simulink model "ECM_EKF_WLTP_kalman"  (R2021b)
settings: Solver=FixedStepDiscrete  StartTime=0.0  StopTime=100000  FixedStep=Ts_data  RelTol=1e-3
PreLoadFcn:
  | % PreLoadFcn — add repo root to MATLAB path before model loads
  | try
  |     mdlName = bdroot;
  |     mdlFile = get_param(mdlName,'FileName');
  |     mdlDir  = fileparts(mdlFile);
  |     repoRoot = fileparts(mdlDir);
  | 
  | 
  |     addpath(genpath(repoRoot));
  |     cd(repoRoot);   % ensure relative paths work while loading
  | catch ME
  |     warning('PreLoadFcn path init failed: %s', ME.message);
  | end
PostLoadFcn:
  | % LoadFcn — run scripts after model loads
  | try
  |     setup_ecm;               % 1) create/overwrite data dictionary with LUTs
  |     setup_ekf;               % 2) upsert EKF params into dictionary
  |     Measured_data_import;    % 3) import measured data to base workspace
  |     fprintf('[%s] Auto-init complete.\n', bdroot);
  | catch ME
  |     warning('LoadFcn auto-init failed: %s', ME.message);
  | end
undefined symbols (not defined in the file or in its folder): C1_lut, C2_lut, crate_bp, DiscIntNeverNeededParam, H_min, OCV_dVoc_dSOC, OCV_lut, OCV_SOC_bp, Q_proc, R0_lut, R1_lut, R2_lut, R_meas, SoC0_guess, soc_bp, Ts_data
settings Model: DataDictionary=ecm_dd.sldd  Creator=ahmeds28  LastModifiedBy=ahmeds28

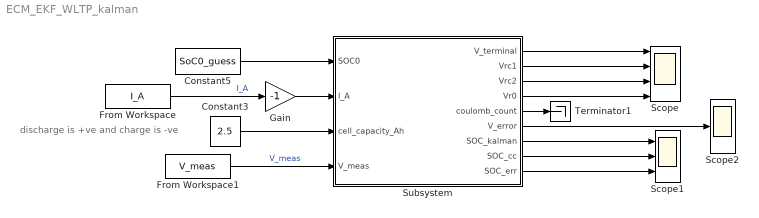
== system ECM_EKF_WLTP_kalman ==
  note: discharge is +ve and charge is -ve
  Constant3 : Constant  Value=2.5
  Constant5 : Constant  Value=SoC0_guess
  From Workspace : FromWorkspace  VariableName=I_A
  From Workspace1 : FromWorkspace  VariableName=V_meas
  Gain : Gain  Gain=-1
  Scope : Scope  NumInputPorts=4
  Scope1 : Scope  NumInputPorts=3
  Scope2 : Scope
  Subsystem : Subsystem
  Terminator1 : Terminator
  wires:
  Constant3/1 -> Subsystem/3(cell_capacity_Ah)
  From Workspace/1 -> Gain/1  "I_A"
  Constant5/1 -> Subsystem/1(SOC0)
  Subsystem/1(V_terminal) -> Scope/1
  Gain/1 -> Subsystem/2(I_A)
  From Workspace1/1 -> Subsystem/4(V_meas)  "V_meas"
  Subsystem/2(Vrc1) -> Scope/2
  Subsystem/3(Vrc2) -> Scope/3
  Subsystem/4(Vr0) -> Scope/4
  Subsystem/7(SOC_kalman) -> Scope1/1
  Subsystem/8(SOC_cc) -> Scope1/2
  Subsystem/9(SOC_err) -> Scope1/3
  Subsystem/6(V_error) -> Scope2/1
  Subsystem/5(coulomb_count) -> Terminator1/1

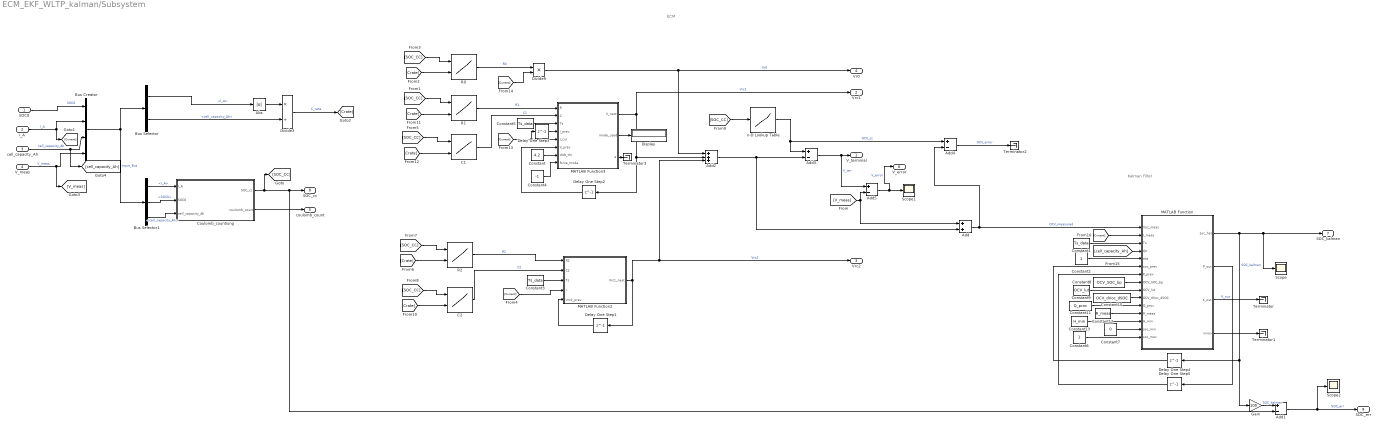
== system ECM_EKF_WLTP_kalman/Subsystem ==
  note: ECM
  note: Kalman Filter
  SOC0 : Inport
  I_A : Inport  Port=2
  cell_capacity_Ah : Inport  Port=3
  V_meas : Inport  Port=4
  Abs : Abs
  Add : Sum
  Add{1,3..5} (4 alike) : Sum  Inputs=+-
  Add2 : Sum  Inputs=+++
  Bus Creator : BusCreator  Inputs=4
  Bus Selector : BusSelector  OutputSignals=I_A,cell_capacity_Ah
  Bus Selector1 : BusSelector  OutputSignals=I_A,SOC0,cell_capacity_Ah
  C1 : Lookup_n-D  LookupTableObject=''  BreakpointsForDimension1=soc_bp  BreakpointsForDimension2=crate_bp  BreakpointsForDimension3=[5, 7]  BreakpointsForDimension1FirstPoint=10  BreakpointsForDimension2FirstPoint=10  BreakpointsForDimension1Spacing=12  BreakpointsForDimension2Spacing=12  IndexSearchMethod=Linear search  Table=C1_lut  InterpMethod=Flat  DiagnosticForOutOfRangeInput=Error  InternalRulePriority=Speed  RndMeth=Simplest  InputSameDT=on
      settings: InputPortMap=u0,u1
  C2 : Lookup_n-D  LookupTableObject=''  BreakpointsForDimension1=soc_bp  BreakpointsForDimension2=crate_bp  BreakpointsForDimension3=[5, 7]  BreakpointsForDimension1FirstPoint=10  BreakpointsForDimension2FirstPoint=10  BreakpointsForDimension1Spacing=12  BreakpointsForDimension2Spacing=12  IndexSearchMethod=Linear search  Table=C2_lut  InterpMethod=Flat  DiagnosticForOutOfRangeInput=Error  InternalRulePriority=Speed  RndMeth=Simplest  InputSameDT=on
      settings: InputPortMap=u0,u1
  Constant : Constant  Value=4.2
  Constant1 : Constant  Value=Ts_data
  Constant10 : Constant  Value=OCV_dVoc_dSOC
  Constant11 : Constant  Value=Q_proc
  Constant12 : Constant  Value=R_meas
  Constant13 : Constant  Value=H_min
  Constant2 : Constant
  Constant3 : Constant  Value=Ts_data
  Constant4 : Constant  Value=-1
  Constant5 : Constant  Value=Ts_data
  Constant6 : Constant
  Constant7 : Constant  Value=0
  Constant8 : Constant  Value=OCV_SOC_bp
  Constant9 : Constant  Value=OCV_lut
  Coulomb_countiung : Subsystem
  Delay One Step1 : Delay  DelayLength=1
  Delay One Step2 : Delay  DelayLength=1
  Delay One Step3 : Delay  DelayLength=1
  Delay One Step4 : Delay  DelayLength=1  InitialCondition=SoC0_guess/100
  Delay One Step5 : Delay  DelayLength=1  InitialCondition=0
  Display : Display
  Divide3 : Product  Inputs=*/
  Divide9 : Product  Inputs=**
  Gain : Gain  Gain=100
  MATLAB Function : MATLAB Function  TreatAsAtomicUnit=on
  MATLAB Function2 : MATLAB Function  TreatAsAtomicUnit=on
  MATLAB Function3 : MATLAB Function  TreatAsAtomicUnit=on
  R0 : Lookup_n-D  LookupTableObject=''  BreakpointsForDimension1=soc_bp  BreakpointsForDimension2=crate_bp  BreakpointsForDimension3=[5, 7]  BreakpointsForDimension1FirstPoint=10  BreakpointsForDimension2FirstPoint=10  BreakpointsForDimension1Spacing=12  BreakpointsForDimension2Spacing=12  IndexSearchMethod=Linear search  Table=R0_lut  InterpMethod=Flat  DiagnosticForOutOfRangeInput=Error  InternalRulePriority=Speed  RndMeth=Simplest  InputSameDT=on
      settings: InputPortMap=u0,u1
  R1 : Lookup_n-D  LookupTableObject=''  BreakpointsForDimension1=soc_bp  BreakpointsForDimension2=crate_bp  BreakpointsForDimension3=[5, 7]  BreakpointsForDimension1FirstPoint=10  BreakpointsForDimension2FirstPoint=10  BreakpointsForDimension1Spacing=12  BreakpointsForDimension2Spacing=12  IndexSearchMethod=Linear search  Table=R1_lut  InterpMethod=Flat  DiagnosticForOutOfRangeInput=Error  InternalRulePriority=Speed  RndMeth=Simplest  InputSameDT=on
      settings: InputPortMap=u0,u1
  R2 : Lookup_n-D  LookupTableObject=''  BreakpointsForDimension1=soc_bp  BreakpointsForDimension2=crate_bp  BreakpointsForDimension3=[5, 7]  BreakpointsForDimension1FirstPoint=10  BreakpointsForDimension2FirstPoint=10  BreakpointsForDimension1Spacing=12  BreakpointsForDimension2Spacing=12  IndexSearchMethod=Linear search  Table=R2_lut  InterpMethod=Flat  DiagnosticForOutOfRangeInput=Error  InternalRulePriority=Speed  RndMeth=Simplest  InputSameDT=on
      settings: InputPortMap=u0,u1
  Scope : Scope
  Scope1 : Scope
  Scope2 : Scope
  Terminator{,1..3} (4 alike) : Terminator
  n-D Lookup Table : Lookup_n-D  NumberOfTableDimensions=1  BreakpointsForDimension1=OCV_SOC_bp  BreakpointsForDimension3=[5, 7]  Table=OCV_lut  InternalRulePriority=Speed  RndMeth=Simplest  InputSameDT=on
  V_terminal : Outport
  Vrc1 : Outport  Port=2
  Vrc2 : Outport  Port=3
  Vr0 : Outport  Port=4
  coulomb_count : Outport  Port=5
  V_error : Outport  Port=6
  SOC_kalman : Outport  Port=7
  SOC_cc : Outport  Port=8
  SOC_err : Outport  Port=9
  wires:
  Bus Selector/1 -> Abs/1  "<I_A>"
  Bus Selector/2 -> Divide3/2  "<cell_capacity_Ah>"
  Divide3/1 -> [Crate]  "C_rate"
  Abs/1 -> Divide3/1
  [Crate] -> R0/2
  [SOC_CC] -> R0/1
  [Crate] -> R2/2
  [SOC_CC] -> R2/1
  [Crate] -> C2/2
  [SOC_CC] -> C2/1
  R0/1 -> Divide9/1  "R0"
  [Current] -> Divide9/2
  Divide9/1 -> Vr0/1, Add2/1  "Vr0"
  [SOC_CC] -> n-D Lookup Table/1
  n-D Lookup Table/1 -> Add4/1, Add3/1  "OCV_cc"
  Add2/1 -> Add/2, Add3/2
  Add3/1 -> Add5/1, V_terminal/1  "V_ter"
  [Crate] -> R1/2
  [SOC_CC] -> C1/1
  [Crate] -> C1/2
  R1/1 -> MATLAB Function3/1(R)  "R1"
  C1/1 -> MATLAB Function3/2(C)  "C1"
  [SOC_CC] -> R1/1
  [Current] -> Delay One Step3/1, MATLAB Function3/5(I_cur)
  MATLAB Function3/1(V_next) -> Add2/2, Delay One Step2/1, Vrc1/1  "Vrc1"
  Constant5/1 -> MATLAB Function3/3(Ts)
  Delay One Step1/1 -> MATLAB Function2/5(Vrc2_prev)
  [Current] -> MATLAB Function2/4(I)
  MATLAB Function2/1(Vrc1_next) -> Vrc2/1, Add2/3, Delay One Step1/1  "Vrc2"
  C2/1 -> MATLAB Function2/2(C2)  "C2"
  Constant3/1 -> MATLAB Function2/3(Ts)
  R2/1 -> MATLAB Function2/1(R2)  "R2"
  Delay One Step2/1 -> MATLAB Function3/6(V_prev)
  Delay One Step3/1 -> MATLAB Function3/4(I_prev)
  MATLAB Function3/2(mode_used) -> Display/1
  Constant/1 -> MATLAB Function3/7(dIdt_thr)
  Constant4/1 -> MATLAB Function3/8(force_mode)
  I_A/1 -> [Current], Bus Creator/2  "I_A"
  SOC0/1 -> Bus Creator/1  "SOC0"
  cell_capacity_Ah/1 -> [cell_capacity_Ah], Bus Creator/3  "cell_capacity_Ah"
  Coulomb_countiung/2(coulomb_count) -> coulomb_count/1
  Bus Creator/1 -> Bus Selector1/1, Bus Selector/1  "Input_Bus"
  Bus Selector1/1 -> Coulomb_countiung/1(I_A)  "<I_A>"
  Bus Selector1/3 -> Coulomb_countiung/3(cell_capacity_Ah)  "<cell_capacity_Ah>"
  Bus Selector1/2 -> Coulomb_countiung/2(SOC0)  "<SOC0>"
  Add5/1 -> V_error/1, Scope1/1  "V_error"
  V_meas/1 -> [V_meas], Bus Creator/4  "V_meas"
  [V_meas] -> Add5/2, Add/1
  Add/1 -> Add4/2, MATLAB Function/1(Voc_meas)  "OCV_measured"
  MATLAB Function/1(soc_hat) -> Delay One Step4/1, Gain/1, Scope/1, SOC_kalman/1  "SOC_kalman"
  Delay One Step4/1 -> MATLAB Function/6(soc_prev)
  MATLAB Function/2(P_out) -> Delay One Step5/1
  Delay One Step5/1 -> MATLAB Function/7(P_prev)
  Constant2/1 -> MATLAB Function/5(eta)
  [cell_capacity_Ah] -> MATLAB Function/4(Qn)
  Constant1/1 -> MATLAB Function/3(Ts)
  [Current] -> MATLAB Function/2(I_meas)
  Coulomb_countiung/1(SOC_cc) -> [SOC_CC], Add1/2, SOC_cc/1
  Add1/1 -> Scope2/1, SOC_err/1  "SOC_err"
  Constant6/1 -> MATLAB Function/15(soc_max)
  Constant7/1 -> MATLAB Function/14(soc_min)
  Constant8/1 -> MATLAB Function/8(OCV_SOC_bp)
  Constant9/1 -> MATLAB Function/9(OCV_lut)
  Constant10/1 -> MATLAB Function/10(OCV_dVoc_dSOC)
  Constant11/1 -> MATLAB Function/11(Q_proc)
  Constant12/1 -> MATLAB Function/12(R_meas)
  Constant13/1 -> MATLAB Function/13(H_min)
  Gain/1 -> Add1/1  "SOC_kalman"
  Add4/1 -> Terminator2/1  "OCV_error"
  MATLAB Function/3(K_out) -> Terminator/1  "K_out"
  MATLAB Function/4(innov) -> Terminator1/1
  MATLAB Function3/3(a) -> Terminator3/1

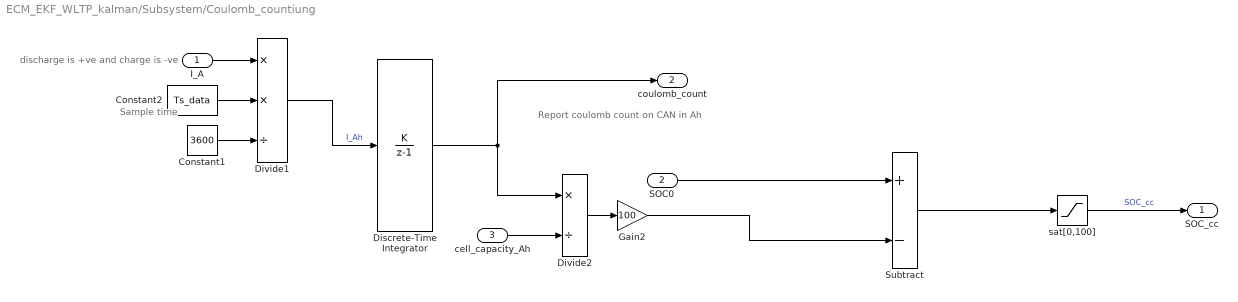
== system ECM_EKF_WLTP_kalman/Subsystem/Coulomb_countiung ==
  note: discharge is +ve and charge is -ve
  note: Report coulomb count on CAN in Ah
  note: Sample time
  I_A : Inport
  SOC0 : Inport  Port=2
  cell_capacity_Ah : Inport  Port=3
  Constant1 : Constant  Value=3600
  Constant2 : Constant  Value=Ts_data
  Discrete-Time Integrator : DiscreteIntegrator  IntegratorMethod=Accumulation: Forward Euler  SampleTime=-1  LimitOutput=on  UpperSaturationLimit=175000  LowerSaturationLimit=-175000  ICPrevOutput=DiscIntNeverNeededParam  ICPrevScaledInput=DiscIntNeverNeededParam
      settings: AttributesFormatString=|
      | %<UpperSaturationLimit>
      | %<LowerSaturationLimit>
  Divide1 : Product  Inputs=**/
  Divide2 : Product  Inputs=*/
  Gain2 : Gain  Gain=100
  Subtract : Sum  Inputs=+-
  sat[0,100] : Saturate  UpperLimit=100  LowerLimit=0
  SOC_cc : Outport
  coulomb_count : Outport  Port=2
  wires:
  Divide1/1 -> Discrete-Time Integrator/1  "I_Ah"
  sat[0,100]/1 -> SOC_cc/1  "SOC_cc"
  Discrete-Time Integrator/1 -> coulomb_count/1, Divide2/1
  cell_capacity_Ah/1 -> Divide2/2
  Constant2/1 -> Divide1/2
  I_A/1 -> Divide1/1
  Divide2/1 -> Gain2/1
  Gain2/1 -> Subtract/2
  Subtract/1 -> sat[0,100]/1
  Constant1/1 -> Divide1/3
  SOC0/1 -> Subtract/1

== matlab function ECM_EKF_WLTP_kalman/Subsystem/MATLAB Function ==
  data: Voc_meas input; soc_hat output; I_meas input; Ts input; Qn input; eta input; soc_prev input; P_prev input; P_out output; K_out output; innov output; OCV_SOC_bp input; OCV_lut input; OCV_dVoc_dSOC input; Q_proc input; R_meas input; H_min input; soc_min input; soc_max input

function [soc_hat, P_out, K_out, innov] = soc_ekf_A_dd( ...
    Voc_meas, I_meas, Ts, Qn, eta, ...
    soc_prev, P_prev, ...
    OCV_SOC_bp, OCV_lut, OCV_dVoc_dSOC, ...
    Q_proc, R_meas, H_min, soc_min, soc_max)
% Hardened voltage-domain SOC EKF (Path-B).
% - Prefers prediction in pulses & OCV plateaus via R scheduling
% - NIS gating to skip outliers/transients
% - Trust region (±1% SOC/step) on correction to avoid jumps
% - Joseph-stabilized covariance (keeps P >= 0)
%
% Inputs (all via block ports; Option-A style):
%   Voc_meas       : de-polarized voltage [V] = V + v1 + v2 + R0*I_meas
%   I_meas         : current [A], discharge-positive convention
%   Ts             : sample time [s]
%   Qn             : nominal capacity [Ah]
%   eta            : Coulombic efficiency [0..1] (use 1.0 if you decided so)
%   soc_prev       : previous SOC estimate [0..1]
%   P_prev         : previous SOC covariance
%   OCV_SOC_bp     : [%] SOC breakpoints (strictly increasing), vector
%   OCV_lut        : [V] OCV values aligned with OCV_SOC_bp, vector
%   OCV_dVoc_dSOC  : [V per fractional SOC], aligned with OCV_SOC_bp, vector
%   Q_proc         : SOC process variance (per-step) [scalar]
%   R_meas         : base voltage measurement variance [scalar, V^2]
%   H_min          : minimum Jacobian (slope floor) [scalar, V/SOC]
%   soc_min/max    : clamp bounds [scalar]
%
% Outputs:
%   soc_hat        : updated SOC estimate
%   P_out          : updated SOC covariance (Joseph-stabilized)
%   K_out          : scalar Kalman gain (voltage-domain)
%   innov          : voltage innovation (Voc_meas - OCV(soc_pred))

% ----------------------------
% 0) Tunables for Path-B logic
% ----------------------------

alpha_R        = 0.10;   % inflate R with |I| (0.08–0.15 typical for “ignore measurement”)
alpha_plateau  = 2.0;    % inflate R when slope is small (1.5–3.0)
H_ref          = 0.03;   % reference slope [V per fractional SOC] (0.03–0.05)
nis_gate       = 2.71;   % ~90% chi-square gate (reject more often than 95%)
delta_cap      = 0.005;  % trust region: limit per-step SOC correction to ±0.5%

% ----------------------------
% 1) Prediction (coulomb count)
% ----------------------------
% NOTE: Qn in Ah -> convert via / (Qn*3600). With discharge-positive current,
% SOC must decrease under discharge.
soc_pred = soc_prev - (eta * Ts * I_meas) / (Qn * 3600);
soc_pred = min(max(soc_pred, soc_min), soc_max);

% If Q_proc is per-step, use as-is. If per-second, use Q_proc*Ts.
P_pred = P_prev + Q_proc;

% ----------------------------
% 2) OCV & slope lookup
% ----------------------------
% Convert breakpoints from percent to fractional SOC and clamp lookup
bp_frac = OCV_SOC_bp(:) / 100;    % [N x 1], fractional SOC
voc_tab = OCV_lut(:);             % [N x 1]
dH_tab  = OCV_dVoc_dSOC(:);       % [N x 1], V per fractional SOC

% Clamp SOC to the table's range for interpolation (avoid extrap artifacts)
soc_q = min(max(soc_pred, bp_frac(1)), bp_frac(end));

% 'linear' is MATLAB Function/codegen-safe; if sim-only, you may switch to 'pchip'
Voc_pred  = interp1(bp_frac, voc_tab, soc_q, 'linear');        % predicted voltage
dVoc_dSOC = interp1(bp_frac, dH_tab,  soc_q, 'linear');        % Jacobian (slope)

% Guard the slope
if ~isfinite(dVoc_dSOC)
    H = H_min;
else
    H = max(dVoc_dSOC, H_min);   % numerical floor only
end

% ----------------------------
% 3) R scheduling (prefer prediction in pulses & plateaus)
% ----------------------------
% Inflate measurement variance when |I| is large and when OCV slope is small.
R_eff = R_meas * (1 + alpha_R * abs(I_meas)) * (1 + alpha_plateau * (H_ref / H)^2);

% ----------------------------
% 4) Innovation, gain, gating
% ----------------------------
innov = Voc_meas - Voc_pred;              % voltage innovation, z - z_hat

S = H*H*P_pred + R_eff;                   % scalar innovation variance
if S < 1e-12, S = 1e-12; end

K = (P_pred * H) / S;                     % voltage-domain gain

% NIS gating (skip update when innovation is statistically unlikely)
NIS = (innov * innov) / S;                % chi-square, 1 dof
if NIS > nis_gate
    K = 0.0;                              % trust prediction only this sample
end

% ----------------------------
% 5) Update with trust region
% ----------------------------
delta  = K * innov;                       % SOC correction (via voltage-domain gain)
% Limit correction to ±delta_cap per step to avoid large jumps
if delta >  delta_cap, delta =  delta_cap; end
if delta < -delta_cap, delta = -delta_cap; end

soc_hat = soc_pred + delta;
soc_hat = min(max(soc_hat, soc_min), soc_max);

% Jocobian-stabilized covariance (keeps P non-negative), using R_eff
P_out = (1 - K*H)^2 * P_pred + (K*K) * R_eff;

K_out = K;  % for logging/tuning
end

== matlab function ECM_EKF_WLTP_kalman/Subsystem/MATLAB Function2 ==
  data: R2 input; Vrc1_next output; C2 input; Ts input; I input; Vrc2_prev input
function Vrc1_next = Vrc2_ZOH(R2, C2, Ts, I, Vrc2_prev)
% Exact ZOH update for fast RC branch
% Guards
R2 = min(max(R2, 1e-6), 10);
C2 = min(max(C2, 1e-6), 1e6);

tau1 = R2 * C2;
a    = exp( - Ts / tau1 );
b    = (1 - a) * R2;

Vrc1_next = a * Vrc2_prev + b * I;
end

== matlab function ECM_EKF_WLTP_kalman/Subsystem/MATLAB Function3 ==
  data: R input; V_next output; C input; Ts input; I_prev input; I_cur input; V_prev input; dIdt_thr input; force_mode input; mode_used output; a output

function [V_next, mode_used, a] = Vrc_FOHZOH(R, C, Ts, I_prev, I_cur, V_prev, dIdt_thr, force_mode)
% Hybrid FOH/ZOH update for a single RC branch, without charge-preservation.
% ZOH is exact for staircase inputs; FOH is exact for piecewise-linear ramps.

% ---------- Guards ----------
R  = min(max(R,  1e-6), 10);      % ohm
C  = min(max(C,  1e-6), 1e8);     % F (slow branch can be large)
Ts = max(Ts, 1e-6);               % s
tau = R * C;
a   = exp(-Ts / tau);             % exact decay factor

% ZOH (exact for holds): V[k] = a*V[k-1] + (1-a)*R*I[k-1]
Vzoh = a * V_prev + (1 - a) * R * I_prev;

% FOH (exact for ramps within the sample):
% Coefficients satisfy B_prev + B_cur = R*(1 - a)
B_prev = R - R * (tau/Ts) * (1 - a);
B_cur  = R * (tau/Ts) * (1 - a) - R * a;
Vfoh   = a * V_prev + B_prev * I_prev + B_cur * I_cur;

% ---------- Mode selection with hysteresis ----------
persistent last_mode
if isempty(last_mode), last_mode = 0; end             % start in ZOH
if force_mode == 0
    mode = 0;                                         % force ZOH
elseif force_mode == 1
    mode = 1;                                         % force FOH
else
    dIdt = (I_cur - I_prev) / Ts;
    if last_mode == 0 && abs(dIdt) > dIdt_thr
        mode = 1;                                     % ZOH -> FOH on strong ramp
    elseif last_mode == 1 && abs(dIdt) < 0.7 * dIdt_thr
        mode = 0;                                     % FOH -> ZOH when ramp weakens
    else
        mode = last_mode;                             % hold mode (avoid chatter)
    end
end

% ---------- Output ----------
V_next    = (mode==1) * Vfoh + (mode==0) * Vzoh;
mode_used = mode;
last_mode = mode;

% Optional clamp for sanity
V_next = min(max(V_next, -1e3), 1e3);
end
